simulink library "tqd"  (R2021b)
settings: Solver=VariableStepAuto  StartTime=0.0  StopTime=10.0  RelTol=1e-3
undefined symbols (not defined in the file): ATQD_AfterTqMinGain_X_Deg, ATQD_APSCreepBaseTqD_X_kph, ATQD_APSCreepBaseTqD_Y_Deg, ATQD_APSCreepBaseTqR_X_kph, ATQD_APSCreepBaseTqR_Y_Deg, ATQD_APSCreepIterm_X_kph, ATQD_APSCreepIterm_Y_kph, ATQD_APSCreepPterm_X_kph, ATQD_APSCreepPterm_Y_kph, ATQD_APSDecReq_X_kph, ATQD_APSDecReq_Y_mps2, ATQD_APSDecReqCMD_X_kph, ATQD_APSDecReqTs_X_pct, ATQD_APSDecTimeGain_X_Deg, ATQD_APSDecTimeGain_Y_s, ATQD_APSReqLowSpd_X_Deg, ATQD_AutoHoldReleaseBPS_X_Deg, ATQD_AWDLoadTrqnsGain_X_kg, ATQD_AWDLoadTrqnsGain_Y_pct, ATQD_BOSEnBPSPosn_X_kph, ATQD_BOSMap_X_rpm, ATQD_BOSMap_Y_pct, ATQD_CreepBaseTqD_X_kph, ATQD_CreepBaseTqD_Y_Deg, ATQD_CreepBaseTqR_X_kph, ATQD_CreepBaseTqR_Y_Deg, ATQD_CreepBPSDisPosn_X_Deg, ATQD_CreepBPSDisPosnR_X_Deg, ATQD_CreepBPSEnPosn_X_Deg, ATQD_CreepBPSEnPosnR_X_Deg, ATQD_CreepDeltaTq_X_kph, ATQD_CreepIterm_X_kph, ATQD_CreepIterm_Y_kph, ATQD_CreepItermMaxLimit_X_pct, ATQD_CreepPreloadTime_X_kph, ATQD_CreepPreloadTq_X_kph, ATQD_CreepPreloadTq_Y_s, ATQD_CreepProtTq_X_Deg, ATQD_CreepPterm_X_kph, ATQD_CreepPterm_Y_kph, ATQD_CreepRrTqSpRat_X_rpm, ATQD_CreepRrTqSpRat_Y_Nm, ATQD_CreepTargetSpdD_X_pct, ATQD_CreepTargetSpdR_X_pct, ATQD_ECOTqMapD_X_rpm, ATQD_ECOTqMapD_Y_pct, ATQD_EMTqMapD_X_rpm, ATQD_EMTqMapD_Y_pct, ATQD_EOPDTqMapDCon_X_rpm, ATQD_EOPDTqMapDCon_Y_Deg, ATQD_EscapeModePedTq_X_pct, ATQD_EscapeModePedTq_Y_rpm, ATQD_EscapeModePedTqFr_X_pct, ATQD_EscapeModePedTqFr_Y_rpm, ATQD_EstInitVehWeight_X_c, ATQD_FAfterTqCMDGain_X_rpm, ATQD_FAfterTqCMDGain_Y_pct, ATQD_FrLossMAPLowV_X_rpm, ATQD_FrLossMAPLowV_Y_Nm, ATQD_FrMotActReduce_X_rpm ... (+772)
libraries: simulink x211, hcu_lib x179, tqr x3
(part 20 of 28)

== system tqd/TQD/TorqueDemand/Signal_convert/SWC2_Subsystem/Big Mike Combo/Combo Key Detection/Engineering Mode ==
  note: Engineering Mode:
      | 5 = VINP_SWC2RScrollUpSta_flg
      | 5 = VINP_SWC2RScrollUpSta_flg
      | 6 = VINP_SWC2RScrollDownSta_flg
      | 6 = VINP_SWC2RScrollDownSta_flg
      | 5 = VINP_SWC2RScrollUpSta_flg
      | 6 = VINP_SWC2RScrollDownSta_flg
      | 5 = VINP_SWC2RScrollUpSta_flg
      | 6 = VINP_SWC2RScrollDownSta_flg
  TASK_TIME_10_MS : Inport
  VSCP_ComboKeyEn_flg : Inport  Port=2
  VSCP_ComboKeyReset_flg : Inport  Port=3
  VSCP_ComboKey_enum : Inport  Port=4
  VSCP_ComboKeyEnter_flg : Inport  Port=5
  VSCP_StreetFightModeOff_flg : Inport  Port=6
  AND : Logic  Inputs=9  AllPortsSameDT=off  OutDataTypeStr=boolean
  Constant : Constant  Value=ENUM_COMBOKEY_NONE
  Constant1 : Constant  Value=ENUM_COMBOKEY_NONE
  Constant2 : Constant  Value=FALSE
  Constant3 : Constant  Value=KTQD_ComboKeyDelay_s
  Delay : Delay  DelayLength=1
  DelayEnable : hcu_lib/Basic_Blocks/DelayEnable
  Equal : RelationalOperator  Operator=~=  OutDataTypeStr=boolean  RndMeth=Simplest
  Key1 : Subsystem
  Key2 : Subsystem
  Key3 : Subsystem
  Key4 : Subsystem
  Key5 : Subsystem
  Key6 : Subsystem
  Key7 : Subsystem
  Key8 : Subsystem
  Switch : Switch  Criteria=u2 > Threshold
  Switch1 : Switch  Criteria=u2 > Threshold
  Switch2 : Switch  Criteria=u2 > Threshold
  VSCP_EngineeringMode_flg : Outport
  wires:
  [VSCP_EngineeringMode_flg] -> VSCP_EngineeringMode_flg/1
  Switch/1 -> [VSCP_ComboKeyCMD_enum]  "VTQD_EngineeringCMD_enum"
  [TASK_TIME_10_MS] -> DelayEnable/3
  Constant/1 -> Switch/3
  DelayEnable/1 -> Switch/2
  [VSCP_ComboKeyEn_flg] -> DelayEnable/1
  Constant3/1 -> DelayEnable/2
  [VSCP_ComboKey_enum] -> Switch/1
  [VSCP_ComboKeyCMD_enum] -> Key1/1(VSCP_ComboKeyCMD_enum)
  [VSCP_ComboKeyEn_flg] -> Key1/2(VSCP_ComboKeyEn_flg)
  [VSCP_ComboKeyReset_flg] -> Key1/3(VSCP_ComboKeyReset_flg)
  [VSCP_ComboKeyCMD_enum] -> Key2/1(VSCP_ComboKeyCMD_enum)
  [VSCP_ComboKeyEn_flg] -> Key2/2(VSCP_ComboKeyEn_flg)
  [VSCP_ComboKeyReset_flg] -> Key2/3(VSCP_ComboKeyReset_flg)
  [VSCP_ComboKey1_enum] -> Key2/4(VSCP_ComboKey1_enum)
  Key1/1(VSCP_ComboKey1_enum) -> [VSCP_ComboKey1_enum]
  Key1/2(VSCP_Key1Pass_flg) -> [VSCP_Key1Pass_flg]
  [VSCP_ComboKeyCMD_enum] -> Key3/1(VSCP_ComboKeyCMD_enum)
  [VSCP_ComboKeyEn_flg] -> Key3/2(VSCP_ComboKeyEn_flg)
  [VSCP_ComboKeyReset_flg] -> Key3/3(VSCP_ComboKeyReset_flg)
  [VSCP_ComboKey2_enum] -> Key3/4(VSCP_ComboKey2_enum)
  [VSCP_ComboKeyCMD_enum] -> Key4/1(VSCP_ComboKeyCMD_enum)
  [VSCP_ComboKeyEn_flg] -> Key4/2(VSCP_ComboKeyEn_flg)
  [VSCP_ComboKeyReset_flg] -> Key4/3(VSCP_ComboKeyReset_flg)
  Key2/1(VSCP_ComboKey2_enum) -> [VSCP_ComboKey2_enum]
  Key2/2(VSCP_Key2Pass_flg) -> [VSCP_Key2Pass_flg]
  [VSCP_ComboKey3_enum] -> Key4/4(VSCP_ComboKey3_enum)
  Key3/1(VSCP_ComboKey3_enum) -> [VSCP_ComboKey3_enum]
  Key3/2(VSCP_Key3Pass_flg) -> [VSCP_Key3Pass_flg]
  Key4/1(VSCP_ComboKey4_enum) -> [VSCP_ComboKey4_enum]
  Key4/2(VSCP_Key4Pass_flg) -> [VSCP_Key4Pass_flg]
  [VSCP_ComboKeyReset_flg] -> Key5/3(VSCP_ComboKeyReset_flg)
  [VSCP_ComboKeyEn_flg] -> Key5/2(VSCP_ComboKeyEn_flg)
  [VSCP_ComboKeyCMD_enum] -> Key5/1(VSCP_ComboKeyCMD_enum)
  [VSCP_ComboKey4_enum] -> Key5/4(VSCP_ComboKey4_enum)
  Key5/2(VSCP_Key5Pass_flg) -> [VSCP_Key5Pass_flg]
  Key5/1(VSCP_ComboKey5_enum) -> [VSCP_ComboKey5_enum]
  Key7/2(VSCP_Key7Pass_flg) -> [VSCP_Key7Pass_flg]
  Key8/1(VSCP_ComboKey8_enum) -> [VSCP_ComboKey8_enum]
  Key8/2(VSCP_Key8Pass_flg) -> [VSCP_Key8Pass_flg]
  [VSCP_ComboKeyCMD_enum] -> Key6/1(VSCP_ComboKeyCMD_enum)
  [VSCP_ComboKeyEn_flg] -> Key6/2(VSCP_ComboKeyEn_flg)
  [VSCP_ComboKeyReset_flg] -> Key6/3(VSCP_ComboKeyReset_flg)
  [VSCP_ComboKey5_enum] -> Key6/4(VSCP_ComboKey5_enum)
  [VSCP_ComboKeyCMD_enum] -> Key7/1(VSCP_ComboKeyCMD_enum)
  [VSCP_ComboKeyEn_flg] -> Key7/2(VSCP_ComboKeyEn_flg)
  [VSCP_ComboKeyReset_flg] -> Key7/3(VSCP_ComboKeyReset_flg)
  [VSCP_ComboKey6_enum] -> Key7/4(VSCP_ComboKey6_enum)
  [VSCP_ComboKeyCMD_enum] -> Key8/1(VSCP_ComboKeyCMD_enum)
  [VSCP_ComboKeyEn_flg] -> Key8/2(VSCP_ComboKeyEn_flg)
  [VSCP_ComboKeyReset_flg] -> Key8/3(VSCP_ComboKeyReset_flg)
  [VSCP_ComboKey7_enum] -> Key8/4(VSCP_ComboKey7_enum)
  Constant1/1 -> Equal/2
  Equal/1 -> AND/1
  [VSCP_Key1Pass_flg] -> AND/2
  [VSCP_Key8Pass_flg] -> AND/9
  [VSCP_Key7Pass_flg] -> AND/8
  [VSCP_Key6Pass_flg] -> AND/7
  [VSCP_Key5Pass_flg] -> AND/6
  [VSCP_Key4Pass_flg] -> AND/5
  [VSCP_Key3Pass_flg] -> AND/4
  [VSCP_Key2Pass_flg] -> AND/3
  [VSCP_ComboKeyEnter_flg] -> Switch1/2
  AND/1 -> Switch1/1  "VTQD_EngineeringPass_flg"
  Switch1/1 -> Switch2/3
  [VSCP_StreetFightModeOff_flg] -> Switch2/2
  Constant2/1 -> Switch2/1
  Switch2/1 -> Delay/1, [VSCP_EngineeringMode_flg]  "VTQD_EngineeringMode_flg"
  Delay/1 -> Switch1/3
  TASK_TIME_10_MS/1 -> [TASK_TIME_10_MS]
  VSCP_ComboKeyEn_flg/1 -> [VSCP_ComboKeyEn_flg]
  VSCP_ComboKeyReset_flg/1 -> [VSCP_ComboKeyReset_flg]
  VSCP_ComboKey_enum/1 -> [VSCP_ComboKey_enum]
  VSCP_ComboKeyEnter_flg/1 -> [VSCP_ComboKeyEnter_flg]
  VSCP_StreetFightModeOff_flg/1 -> [VSCP_StreetFightModeOff_flg]
  Key6/1(VSCP_ComboKey6_enum) -> [VSCP_ComboKey6_enum]
  Key6/2(VSCP_Key6Pass_flg) -> [VSCP_Key6Pass_flg]
  Key7/1(VSCP_ComboKey7_enum) -> [VSCP_ComboKey7_enum]
  [VSCP_ComboKey8_enum] -> Equal/1

== system tqd/TQD/TorqueDemand/Signal_convert/SWC2_Subsystem/Big Mike Combo/Combo Key Detection/Exhibition Mode ==
  note: Exhibition Mode:
      | 7 = VINP_SWC2LScrollPressSta_flg
      | 7 = VINP_SWC2LScrollPressSta_flg
      | 8 = VINP_SWC2LADASSta_flg
      | 8 = VINP_SWC2LADASSta_flg
      | 8 = VINP_SWC2LADASSta_flg
      | 7 = VINP_SWC2LScrollPressSta_flg
      | 8 = VINP_SWC2LADASSta_flg
      | 7 = VINP_SWC2LScrollPressSta_flg
  TASK_TIME_10_MS : Inport
  VSCP_ComboKeyEn_flg : Inport  Port=2
  VSCP_ComboKeyReset_flg : Inport  Port=3
  VSCP_ComboKey_enum : Inport  Port=4
  VSCP_ComboKeyEnter_flg : Inport  Port=5
  VSCP_StreetFightModeOff_flg : Inport  Port=6
  AND : Logic  Inputs=9  AllPortsSameDT=off  OutDataTypeStr=boolean
  Constant : Constant  Value=ENUM_COMBOKEY_NONE
  Constant1 : Constant  Value=ENUM_COMBOKEY_NONE
  Constant2 : Constant  Value=FALSE
  Constant3 : Constant  Value=KTQD_ComboKeyDelay_s
  Delay : Delay  DelayLength=1
  DelayEnable : hcu_lib/Basic_Blocks/DelayEnable
  Equal : RelationalOperator  Operator=~=  OutDataTypeStr=boolean  RndMeth=Simplest
  Key1 : Subsystem
  Key2 : Subsystem
  Key3 : Subsystem
  Key4 : Subsystem
  Key5 : Subsystem
  Key6 : Subsystem
  Key7 : Subsystem
  Key8 : Subsystem
  Switch : Switch  Criteria=u2 > Threshold
  Switch1 : Switch  Criteria=u2 > Threshold
  Switch2 : Switch  Criteria=u2 > Threshold
  VSCP_ExhibitionMode_flg : Outport
  wires:
  [VSCP_ExhibitionMode_flg] -> VSCP_ExhibitionMode_flg/1
  Switch/1 -> [VSCP_ComboKeyCMD_enum]  "VTQD_ExhibitionCMD_enum"
  [TASK_TIME_10_MS] -> DelayEnable/3
  Constant/1 -> Switch/3
  DelayEnable/1 -> Switch/2
  [VSCP_ComboKeyEn_flg] -> DelayEnable/1
  Constant3/1 -> DelayEnable/2
  [VSCP_ComboKey_enum] -> Switch/1
  [VSCP_ComboKeyCMD_enum] -> Key1/1(VSCP_ComboKeyCMD_enum)
  [VSCP_ComboKeyEn_flg] -> Key1/2(VSCP_ComboKeyEn_flg)
  [VSCP_ComboKeyReset_flg] -> Key1/3(VSCP_ComboKeyReset_flg)
  [VSCP_ComboKeyCMD_enum] -> Key2/1(VSCP_ComboKeyCMD_enum)
  [VSCP_ComboKeyEn_flg] -> Key2/2(VSCP_ComboKeyEn_flg)
  [VSCP_ComboKeyReset_flg] -> Key2/3(VSCP_ComboKeyReset_flg)
  [VSCP_ComboKey1_enum] -> Key2/4(VSCP_ComboKey1_enum)
  Key1/1(VSCP_ComboKey1_enum) -> [VSCP_ComboKey1_enum]
  Key1/2(VSCP_Key1Pass_flg) -> [VSCP_Key1Pass_flg]
  [VSCP_ComboKeyCMD_enum] -> Key3/1(VSCP_ComboKeyCMD_enum)
  [VSCP_ComboKeyEn_flg] -> Key3/2(VSCP_ComboKeyEn_flg)
  [VSCP_ComboKeyReset_flg] -> Key3/3(VSCP_ComboKeyReset_flg)
  [VSCP_ComboKey2_enum] -> Key3/4(VSCP_ComboKey2_enum)
  [VSCP_ComboKeyCMD_enum] -> Key4/1(VSCP_ComboKeyCMD_enum)
  [VSCP_ComboKeyEn_flg] -> Key4/2(VSCP_ComboKeyEn_flg)
  [VSCP_ComboKeyReset_flg] -> Key4/3(VSCP_ComboKeyReset_flg)
  Key2/1(VSCP_ComboKey2_enum) -> [VSCP_ComboKey2_enum]
  Key2/2(VSCP_Key2Pass_flg) -> [VSCP_Key2Pass_flg]
  [VSCP_ComboKey3_enum] -> Key4/4(VSCP_ComboKey3_enum)
  Key3/1(VSCP_ComboKey3_enum) -> [VSCP_ComboKey3_enum]
  Key3/2(VSCP_Key3Pass_flg) -> [VSCP_Key3Pass_flg]
  Key4/1(VSCP_ComboKey4_enum) -> [VSCP_ComboKey4_enum]
  Key4/2(VSCP_Key4Pass_flg) -> [VSCP_Key4Pass_flg]
  [VSCP_ComboKeyReset_flg] -> Key5/3(VSCP_ComboKeyReset_flg)
  [VSCP_ComboKeyEn_flg] -> Key5/2(VSCP_ComboKeyEn_flg)
  [VSCP_ComboKeyCMD_enum] -> Key5/1(VSCP_ComboKeyCMD_enum)
  [VSCP_ComboKey4_enum] -> Key5/4(VSCP_ComboKey4_enum)
  Key5/2(VSCP_Key5Pass_flg) -> [VSCP_Key5Pass_flg]
  Key5/1(VSCP_ComboKey5_enum) -> [VSCP_ComboKey5_enum]
  Key7/2(VSCP_Key7Pass_flg) -> [VSCP_Key7Pass_flg]
  Key8/1(VSCP_ComboKey8_enum) -> [VSCP_ComboKey8_enum]
  Key8/2(VSCP_Key8Pass_flg) -> [VSCP_Key8Pass_flg]
  [VSCP_ComboKeyCMD_enum] -> Key6/1(VSCP_ComboKeyCMD_enum)
  [VSCP_ComboKeyEn_flg] -> Key6/2(VSCP_ComboKeyEn_flg)
  [VSCP_ComboKeyReset_flg] -> Key6/3(VSCP_ComboKeyReset_flg)
  [VSCP_ComboKey5_enum] -> Key6/4(VSCP_ComboKey5_enum)
  [VSCP_ComboKeyCMD_enum] -> Key7/1(VSCP_ComboKeyCMD_enum)
  [VSCP_ComboKeyEn_flg] -> Key7/2(VSCP_ComboKeyEn_flg)
  [VSCP_ComboKeyReset_flg] -> Key7/3(VSCP_ComboKeyReset_flg)
  [VSCP_ComboKey6_enum] -> Key7/4(VSCP_ComboKey6_enum)
  [VSCP_ComboKeyCMD_enum] -> Key8/1(VSCP_ComboKeyCMD_enum)
  [VSCP_ComboKeyEn_flg] -> Key8/2(VSCP_ComboKeyEn_flg)
  [VSCP_ComboKeyReset_flg] -> Key8/3(VSCP_ComboKeyReset_flg)
  [VSCP_ComboKey7_enum] -> Key8/4(VSCP_ComboKey7_enum)
  Constant1/1 -> Equal/2
  Equal/1 -> AND/1
  [VSCP_Key1Pass_flg] -> AND/2
  [VSCP_Key8Pass_flg] -> AND/9
  [VSCP_Key7Pass_flg] -> AND/8
  [VSCP_Key6Pass_flg] -> AND/7
  [VSCP_Key5Pass_flg] -> AND/6
  [VSCP_Key4Pass_flg] -> AND/5
  [VSCP_Key3Pass_flg] -> AND/4
  [VSCP_Key2Pass_flg] -> AND/3
  [VSCP_ComboKeyEnter_flg] -> Switch1/2
  AND/1 -> Switch1/1  "VTQD_ExhibitionPass_flg"
  Switch1/1 -> Switch2/3
  [VSCP_StreetFightModeOff_flg] -> Switch2/2
  Constant2/1 -> Switch2/1
  Switch2/1 -> Delay/1, [VSCP_ExhibitionMode_flg]  "VTQD_ExhibitionMode_flg"
  Delay/1 -> Switch1/3
  TASK_TIME_10_MS/1 -> [TASK_TIME_10_MS]
  VSCP_ComboKeyEn_flg/1 -> [VSCP_ComboKeyEn_flg]
  VSCP_ComboKeyReset_flg/1 -> [VSCP_ComboKeyReset_flg]
  VSCP_ComboKey_enum/1 -> [VSCP_ComboKey_enum]
  VSCP_ComboKeyEnter_flg/1 -> [VSCP_ComboKeyEnter_flg]
  VSCP_StreetFightModeOff_flg/1 -> [VSCP_StreetFightModeOff_flg]
  Key6/1(VSCP_ComboKey6_enum) -> [VSCP_ComboKey6_enum]
  Key6/2(VSCP_Key6Pass_flg) -> [VSCP_Key6Pass_flg]
  Key7/1(VSCP_ComboKey7_enum) -> [VSCP_ComboKey7_enum]
  [VSCP_ComboKey8_enum] -> Equal/1

== system tqd/TQD/TorqueDemand/Signal_convert/SWC2_Subsystem/Big Mike Combo/Combo Key Detection/Manufacture Mode ==
  note: Manufacture Mode:
      | 11 = VINP_SWC2RRightSta_flg
      | 12 = VINP_SWC2RLeftSta_flg
      | 11 = VINP_SWC2RRightSta_flg
      | 12 = VINP_SWC2RLeftSta_flg
      | 11 = VINP_SWC2RRightSta_flg
      | 12 = VINP_SWC2RLeftSta_flg
      | 7 = VINP_SWC2LScrollPressSta_flg
      | 8 = VINP_SWC2LADASSta_flg
  TASK_TIME_10_MS : Inport
  VSCP_ComboKeyEn_flg : Inport  Port=2
  VSCP_ComboKeyReset_flg : Inport  Port=3
  VSCP_ComboKey_enum : Inport  Port=4
  VSCP_ComboKeyEnter_flg : Inport  Port=5
  VSCP_StreetFightModeOff_flg : Inport  Port=6
  AND : Logic  Inputs=9  AllPortsSameDT=off  OutDataTypeStr=boolean
  Constant : Constant  Value=ENUM_COMBOKEY_NONE
  Constant1 : Constant  Value=ENUM_COMBOKEY_NONE
  Constant2 : Constant  Value=FALSE
  Constant3 : Constant  Value=KTQD_ComboKeyDelay_s
  Delay : Delay  DelayLength=1
  DelayEnable : hcu_lib/Basic_Blocks/DelayEnable
  Equal : RelationalOperator  Operator=~=  OutDataTypeStr=boolean  RndMeth=Simplest
  Key1 : Subsystem
  Key2 : Subsystem
  Key3 : Subsystem
  Key4 : Subsystem
  Key5 : Subsystem
  Key6 : Subsystem
  Key7 : Subsystem
  Key8 : Subsystem
  Switch : Switch  Criteria=u2 > Threshold
  Switch1 : Switch  Criteria=u2 > Threshold
  Switch2 : Switch  Criteria=u2 > Threshold
  VSCP_ManufactureMode_flg : Outport
  wires:
  [VSCP_ComboKey8_enum] -> Equal/1
  Key7/1(VSCP_ComboKey7_enum) -> [VSCP_ComboKey7_enum]
  Key6/2(VSCP_Key6Pass_flg) -> [VSCP_Key6Pass_flg]
  Key6/1(VSCP_ComboKey6_enum) -> [VSCP_ComboKey6_enum]
  VSCP_StreetFightModeOff_flg/1 -> [VSCP_StreetFightModeOff_flg]
  VSCP_ComboKeyEnter_flg/1 -> [VSCP_ComboKeyEnter_flg]
  VSCP_ComboKey_enum/1 -> [VSCP_ComboKey_enum]
  VSCP_ComboKeyReset_flg/1 -> [VSCP_ComboKeyReset_flg]
  VSCP_ComboKeyEn_flg/1 -> [VSCP_ComboKeyEn_flg]
  TASK_TIME_10_MS/1 -> [TASK_TIME_10_MS]
  Delay/1 -> Switch1/3
  Switch2/1 -> [VSCP_ManufactureMode_flg], Delay/1  "VTQD_ManufactureMode_flg"
  Constant2/1 -> Switch2/1
  [VSCP_StreetFightModeOff_flg] -> Switch2/2
  Switch1/1 -> Switch2/3
  AND/1 -> Switch1/1  "VTQD_ManufacturePass_flg"
  [VSCP_ComboKeyEnter_flg] -> Switch1/2
  [VSCP_Key2Pass_flg] -> AND/3
  [VSCP_Key3Pass_flg] -> AND/4
  [VSCP_Key4Pass_flg] -> AND/5
  [VSCP_Key5Pass_flg] -> AND/6
  [VSCP_Key6Pass_flg] -> AND/7
  [VSCP_Key7Pass_flg] -> AND/8
  [VSCP_Key8Pass_flg] -> AND/9
  [VSCP_Key1Pass_flg] -> AND/2
  Equal/1 -> AND/1
  Constant1/1 -> Equal/2
  [VSCP_ComboKey7_enum] -> Key8/4(VSCP_ComboKey7_enum)
  [VSCP_ComboKeyReset_flg] -> Key8/3(VSCP_ComboKeyReset_flg)
  [VSCP_ComboKeyEn_flg] -> Key8/2(VSCP_ComboKeyEn_flg)
  [VSCP_ComboKeyCMD_enum] -> Key8/1(VSCP_ComboKeyCMD_enum)
  [VSCP_ComboKey6_enum] -> Key7/4(VSCP_ComboKey6_enum)
  [VSCP_ComboKeyReset_flg] -> Key7/3(VSCP_ComboKeyReset_flg)
  [VSCP_ComboKeyEn_flg] -> Key7/2(VSCP_ComboKeyEn_flg)
  [VSCP_ComboKeyCMD_enum] -> Key7/1(VSCP_ComboKeyCMD_enum)
  [VSCP_ComboKey5_enum] -> Key6/4(VSCP_ComboKey5_enum)
  [VSCP_ComboKeyReset_flg] -> Key6/3(VSCP_ComboKeyReset_flg)
  [VSCP_ComboKeyEn_flg] -> Key6/2(VSCP_ComboKeyEn_flg)
  [VSCP_ComboKeyCMD_enum] -> Key6/1(VSCP_ComboKeyCMD_enum)
  Key8/2(VSCP_Key8Pass_flg) -> [VSCP_Key8Pass_flg]
  Key8/1(VSCP_ComboKey8_enum) -> [VSCP_ComboKey8_enum]
  Key7/2(VSCP_Key7Pass_flg) -> [VSCP_Key7Pass_flg]
  Key5/1(VSCP_ComboKey5_enum) -> [VSCP_ComboKey5_enum]
  Key5/2(VSCP_Key5Pass_flg) -> [VSCP_Key5Pass_flg]
  [VSCP_ComboKey4_enum] -> Key5/4(VSCP_ComboKey4_enum)
  [VSCP_ComboKeyCMD_enum] -> Key5/1(VSCP_ComboKeyCMD_enum)
  [VSCP_ComboKeyEn_flg] -> Key5/2(VSCP_ComboKeyEn_flg)
  [VSCP_ComboKeyReset_flg] -> Key5/3(VSCP_ComboKeyReset_flg)
  Key4/2(VSCP_Key4Pass_flg) -> [VSCP_Key4Pass_flg]
  Key4/1(VSCP_ComboKey4_enum) -> [VSCP_ComboKey4_enum]
  Key3/2(VSCP_Key3Pass_flg) -> [VSCP_Key3Pass_flg]
  Key3/1(VSCP_ComboKey3_enum) -> [VSCP_ComboKey3_enum]
  [VSCP_ComboKey3_enum] -> Key4/4(VSCP_ComboKey3_enum)
  Key2/2(VSCP_Key2Pass_flg) -> [VSCP_Key2Pass_flg]
  Key2/1(VSCP_ComboKey2_enum) -> [VSCP_ComboKey2_enum]
  [VSCP_ComboKeyReset_flg] -> Key4/3(VSCP_ComboKeyReset_flg)
  [VSCP_ComboKeyEn_flg] -> Key4/2(VSCP_ComboKeyEn_flg)
  [VSCP_ComboKeyCMD_enum] -> Key4/1(VSCP_ComboKeyCMD_enum)
  [VSCP_ComboKey2_enum] -> Key3/4(VSCP_ComboKey2_enum)
  [VSCP_ComboKeyReset_flg] -> Key3/3(VSCP_ComboKeyReset_flg)
  [VSCP_ComboKeyEn_flg] -> Key3/2(VSCP_ComboKeyEn_flg)
  [VSCP_ComboKeyCMD_enum] -> Key3/1(VSCP_ComboKeyCMD_enum)
  Key1/2(VSCP_Key1Pass_flg) -> [VSCP_Key1Pass_flg]
  Key1/1(VSCP_ComboKey1_enum) -> [VSCP_ComboKey1_enum]
  [VSCP_ComboKey1_enum] -> Key2/4(VSCP_ComboKey1_enum)
  [VSCP_ComboKeyReset_flg] -> Key2/3(VSCP_ComboKeyReset_flg)
  [VSCP_ComboKeyEn_flg] -> Key2/2(VSCP_ComboKeyEn_flg)
  [VSCP_ComboKeyCMD_enum] -> Key2/1(VSCP_ComboKeyCMD_enum)
  [VSCP_ComboKeyReset_flg] -> Key1/3(VSCP_ComboKeyReset_flg)
  [VSCP_ComboKeyEn_flg] -> Key1/2(VSCP_ComboKeyEn_flg)
  [VSCP_ComboKeyCMD_enum] -> Key1/1(VSCP_ComboKeyCMD_enum)
  [VSCP_ComboKey_enum] -> Switch/1
  Constant3/1 -> DelayEnable/2
  [VSCP_ComboKeyEn_flg] -> DelayEnable/1
  DelayEnable/1 -> Switch/2
  Constant/1 -> Switch/3
  [TASK_TIME_10_MS] -> DelayEnable/3
  Switch/1 -> [VSCP_ComboKeyCMD_enum]  "VTQD_ManufactureCMD_enum"
  [VSCP_ManufactureMode_flg] -> VSCP_ManufactureMode_flg/1

== system tqd/TQD/TorqueDemand/Signal_convert/SWC2_Subsystem/Big Mike Combo/Combo Key Detection/Street Fight Mode ==
  note: Street Fight Mode:
      | 3 = VINP_SWC2LScrollUpSta_flg
      | 3 = VINP_SWC2LScrollUpSta_flg
      | 4 = VINP_SWC2LScrollDownSta_flg
      | 4 = VINP_SWC2LScrollDownSta_flg
      | 1 = VINP_SWC2RegenDown_flg
      | 1 = VINP_SWC2RegenDown_flg
      | 2 = VINP_SWC2RegenUp_flg
      | 2 = VINP_SWC2RegenUp_flg
  TASK_TIME_10_MS : Inport
  VSCP_ComboKeyEn_flg : Inport  Port=2
  VSCP_ComboKeyReset_flg : Inport  Port=3
  VSCP_ComboKey_enum : Inport  Port=4
  VSCP_ComboKeyEnter_flg : Inport  Port=5
  VSCP_StreetFightModeOff_flg : Inport  Port=6
  AND : Logic  Inputs=9  AllPortsSameDT=off  OutDataTypeStr=boolean
  Constant : Constant  Value=ENUM_COMBOKEY_NONE
  Constant1 : Constant  Value=ENUM_COMBOKEY_NONE
  Constant2 : Constant  Value=FALSE
  Constant3 : Constant  Value=KTQD_ComboKeyDelay_s
  Delay : Delay  DelayLength=1
  DelayEnable : hcu_lib/Basic_Blocks/DelayEnable
  Equal : RelationalOperator  Operator=~=  OutDataTypeStr=boolean  RndMeth=Simplest
  Key1 : Subsystem
  Key2 : Subsystem
  Key3 : Subsystem
  Key4 : Subsystem
  Key5 : Subsystem
  Key6 : Subsystem
  Key7 : Subsystem
  Key8 : Subsystem
  Switch : Switch  Criteria=u2 > Threshold
  Switch1 : Switch  Criteria=u2 > Threshold
  Switch2 : Switch  Criteria=u2 > Threshold
  VSCP_StreetFightMode_flg : Outport
  wires:
  [VSCP_ComboKey8_enum] -> Equal/1
  Key7/1(VSCP_ComboKey7_enum) -> [VSCP_ComboKey7_enum]
  Key6/2(VSCP_Key6Pass_flg) -> [VSCP_Key6Pass_flg]
  Key6/1(VSCP_ComboKey6_enum) -> [VSCP_ComboKey6_enum]
  [VSCP_StreetFightMode_flg] -> VSCP_StreetFightMode_flg/1
  VSCP_StreetFightModeOff_flg/1 -> [VSCP_StreetFightModeOff_flg]
  VSCP_ComboKeyEnter_flg/1 -> [VSCP_ComboKeyEnter_flg]
  VSCP_ComboKey_enum/1 -> [VSCP_ComboKey_enum]
  VSCP_ComboKeyReset_flg/1 -> [VSCP_ComboKeyReset_flg]
  VSCP_ComboKeyEn_flg/1 -> [VSCP_ComboKeyEn_flg]
  TASK_TIME_10_MS/1 -> [TASK_TIME_10_MS]
  Delay/1 -> Switch1/3
  Switch2/1 -> [VSCP_StreetFightMode_flg], Delay/1  "VTQD_StreetFightMode_flg"
  Constant2/1 -> Switch2/1
  [VSCP_StreetFightModeOff_flg] -> Switch2/2
  Switch1/1 -> Switch2/3
  AND/1 -> Switch1/1  "VTQD_StreetFightPass_flg"
  [VSCP_ComboKeyEnter_flg] -> Switch1/2
  [VSCP_Key2Pass_flg] -> AND/3
  [VSCP_Key3Pass_flg] -> AND/4
  [VSCP_Key4Pass_flg] -> AND/5
  [VSCP_Key5Pass_flg] -> AND/6
  [VSCP_Key6Pass_flg] -> AND/7
  [VSCP_Key7Pass_flg] -> AND/8
  [VSCP_Key8Pass_flg] -> AND/9
  [VSCP_Key1Pass_flg] -> AND/2
  Equal/1 -> AND/1
  Constant1/1 -> Equal/2
  [VSCP_ComboKey7_enum] -> Key8/4(VSCP_ComboKey7_enum)
  [VSCP_ComboKeyReset_flg] -> Key8/3(VSCP_ComboKeyReset_flg)
  [VSCP_ComboKeyEn_flg] -> Key8/2(VSCP_ComboKeyEn_flg)
  [VSCP_ComboKeyCMD_enum] -> Key8/1(VSCP_ComboKeyCMD_enum)
  [VSCP_ComboKey6_enum] -> Key7/4(VSCP_ComboKey6_enum)
  [VSCP_ComboKeyReset_flg] -> Key7/3(VSCP_ComboKeyReset_flg)
  [VSCP_ComboKeyEn_flg] -> Key7/2(VSCP_ComboKeyEn_flg)
  [VSCP_ComboKeyCMD_enum] -> Key7/1(VSCP_ComboKeyCMD_enum)
  [VSCP_ComboKey5_enum] -> Key6/4(VSCP_ComboKey5_enum)
  [VSCP_ComboKeyReset_flg] -> Key6/3(VSCP_ComboKeyReset_flg)
  [VSCP_ComboKeyEn_flg] -> Key6/2(VSCP_ComboKeyEn_flg)
  [VSCP_ComboKeyCMD_enum] -> Key6/1(VSCP_ComboKeyCMD_enum)
  Key8/2(VSCP_Key8Pass_flg) -> [VSCP_Key8Pass_flg]
  Key8/1(VSCP_ComboKey8_enum) -> [VSCP_ComboKey8_enum]
  Key7/2(VSCP_Key7Pass_flg) -> [VSCP_Key7Pass_flg]
  Key5/1(VSCP_ComboKey5_enum) -> [VSCP_ComboKey5_enum]
  Key5/2(VSCP_Key5Pass_flg) -> [VSCP_Key5Pass_flg]
  [VSCP_ComboKey4_enum] -> Key5/4(VSCP_ComboKey4_enum)
  [VSCP_ComboKeyCMD_enum] -> Key5/1(VSCP_ComboKeyCMD_enum)
  [VSCP_ComboKeyEn_flg] -> Key5/2(VSCP_ComboKeyEn_flg)
  [VSCP_ComboKeyReset_flg] -> Key5/3(VSCP_ComboKeyReset_flg)
  Key4/2(VSCP_Key4Pass_flg) -> [VSCP_Key4Pass_flg]
  Key4/1(VSCP_ComboKey4_enum) -> [VSCP_ComboKey4_enum]
  Key3/2(VSCP_Key3Pass_flg) -> [VSCP_Key3Pass_flg]
  Key3/1(VSCP_ComboKey3_enum) -> [VSCP_ComboKey3_enum]
  [VSCP_ComboKey3_enum] -> Key4/4(VSCP_ComboKey3_enum)
  Key2/2(VSCP_Key2Pass_flg) -> [VSCP_Key2Pass_flg]
  Key2/1(VSCP_ComboKey2_enum) -> [VSCP_ComboKey2_enum]
  [VSCP_ComboKeyReset_flg] -> Key4/3(VSCP_ComboKeyReset_flg)
  [VSCP_ComboKeyEn_flg] -> Key4/2(VSCP_ComboKeyEn_flg)
  [VSCP_ComboKeyCMD_enum] -> Key4/1(VSCP_ComboKeyCMD_enum)
  [VSCP_ComboKey2_enum] -> Key3/4(VSCP_ComboKey2_enum)
  [VSCP_ComboKeyReset_flg] -> Key3/3(VSCP_ComboKeyReset_flg)
  [VSCP_ComboKeyEn_flg] -> Key3/2(VSCP_ComboKeyEn_flg)
  [VSCP_ComboKeyCMD_enum] -> Key3/1(VSCP_ComboKeyCMD_enum)
  Key1/2(VSCP_Key1Pass_flg) -> [VSCP_Key1Pass_flg]
  Key1/1(VSCP_ComboKey1_enum) -> [VSCP_ComboKey1_enum]
  [VSCP_ComboKey1_enum] -> Key2/4(VSCP_ComboKey1_enum)
  [VSCP_ComboKeyReset_flg] -> Key2/3(VSCP_ComboKeyReset_flg)
  [VSCP_ComboKeyEn_flg] -> Key2/2(VSCP_ComboKeyEn_flg)
  [VSCP_ComboKeyCMD_enum] -> Key2/1(VSCP_ComboKeyCMD_enum)
  [VSCP_ComboKeyReset_flg] -> Key1/3(VSCP_ComboKeyReset_flg)
  [VSCP_ComboKeyEn_flg] -> Key1/2(VSCP_ComboKeyEn_flg)
  [VSCP_ComboKeyCMD_enum] -> Key1/1(VSCP_ComboKeyCMD_enum)
  [VSCP_ComboKey_enum] -> Switch/1
  Constant3/1 -> DelayEnable/2
  [VSCP_ComboKeyEn_flg] -> DelayEnable/1
  DelayEnable/1 -> Switch/2
  Constant/1 -> Switch/3
  [TASK_TIME_10_MS] -> DelayEnable/3
  Switch/1 -> [VSCP_ComboKeyCMD_enum]  "VTQD_StreetFightCMD_enum"

== system tqd/TQD/TorqueDemand/Signal_convert/SWC2_Subsystem/Big Mike Combo/Mode Coordination/DiagnosisOff ==
  Action Port : ActionPort
  Constant : Constant  Value=ENUM_SYSMODE_DIAGNOSISOFF
  DiagnosisOff : Outport
  wires:
  Constant/1 -> DiagnosisOff/1

== system tqd/TQD/TorqueDemand/Signal_convert/SWC2_Subsystem/Big Mike Combo/Mode Coordination/Engineering ==
  Action Port : ActionPort
  Constant : Constant  Value=ENUM_SYSMODE_ENGINEERING
  Engineering : Outport
  wires:
  Constant/1 -> Engineering/1

== system tqd/TQD/TorqueDemand/Signal_convert/SWC2_Subsystem/Big Mike Combo/Mode Coordination/Exhibition ==
  Action Port : ActionPort
  Constant : Constant  Value=ENUM_SYSMODE_EXHIBITION
  Exhibition : Outport
  wires:
  Constant/1 -> Exhibition/1

== system tqd/TQD/TorqueDemand/Signal_convert/SWC2_Subsystem/Big Mike Combo/Mode Coordination/Manufacture ==
  Action Port : ActionPort
  Constant : Constant  Value=ENUM_SYSMODE_MANUFACTURE
  Manufacture : Outport
  wires:
  Constant/1 -> Manufacture/1

== system tqd/TQD/TorqueDemand/Signal_convert/SWC2_Subsystem/Big Mike Combo/Mode Coordination/Product ==
  Action Port : ActionPort
  Constant : Constant  Value=ENUM_SYSMODE_PRODUCT
  Product : Outport
  wires:
  Constant/1 -> Product/1

== system tqd/TQD/TorqueDemand/Signal_convert/SWC2_Subsystem/Big Mike Combo/Mode Coordination/StreetFight ==
  Action Port : ActionPort
  Constant : Constant  Value=ENUM_SYSMODE_DEVELOPING
  StreetFight : Outport
  wires:
  Constant/1 -> StreetFight/1

== system tqd/TQD/TorqueDemand/Signal_convert/SWC2_Subsystem/Big Mike Combo/Signal Status Detection/None ==
  Action Port : ActionPort
  Constant : Constant  Value=ENUM_COMBOKEY_NONE  OutDataTypeStr=uint8
  None_enum : Outport
  wires:
  Constant/1 -> None_enum/1

== system tqd/TQD/TorqueDemand/Signal_convert/SWC2_Subsystem/Big Mike Combo/Signal Status Detection/SWCACCSta ==
  Action Port : ActionPort
  Constant : Constant  Value=ENUM_COMBOKEY_SWCACC  OutDataTypeStr=uint8
  SWCACCSta_enum : Outport
  wires:
  Constant/1 -> SWCACCSta_enum/1

== system tqd/TQD/TorqueDemand/Signal_convert/SWC2_Subsystem/Big Mike Combo/Signal Status Detection/SWCCANCELStaShort ==
  Action Port : ActionPort
  Constant : Constant  Value=ENUM_COMBOKEY_CANCEL  OutDataTypeStr=uint8
  SWCCANCELStaShort_enum : Outport
  wires:
  Constant/1 -> SWCCANCELStaShort_enum/1

== system tqd/TQD/TorqueDemand/Signal_convert/SWC2_Subsystem/Big Mike Combo/Signal Status Detection/SWCDistanceSta ==
  Action Port : ActionPort
  Constant : Constant  Value=ENUM_COMBOKEY_DISTANCE  OutDataTypeStr=uint8
  SWCDownStaShort_enum : Outport
  wires:
  Constant/1 -> SWCDownStaShort_enum/1

== system tqd/TQD/TorqueDemand/Signal_convert/SWC2_Subsystem/Big Mike Combo/Signal Status Detection/SWCDownStaShort ==
  Action Port : ActionPort
  Constant : Constant  Value=ENUM_COMBOKEY_SWCDOWN  OutDataTypeStr=uint8
  SWCDownStaShort_enum : Outport
  wires:
  Constant/1 -> SWCDownStaShort_enum/1

== system tqd/TQD/TorqueDemand/Signal_convert/SWC2_Subsystem/Big Mike Combo/Signal Status Detection/SWCLeftSta ==
  Action Port : ActionPort
  Constant : Constant  Value=ENUM_COMBOKEY_SWCLEFT  OutDataTypeStr=uint8
  SWCLeftSta_enum : Outport
  wires:
  Constant/1 -> SWCLeftSta_enum/1

== system tqd/TQD/TorqueDemand/Signal_convert/SWC2_Subsystem/Big Mike Combo/Signal Status Detection/SWCRegenDownShort ==
  Action Port : ActionPort
  Constant : Constant  Value=ENUM_COMBOKEY_REGENDOWN  OutDataTypeStr=uint8
  SWCRegenDownShort_enum : Outport
  wires:
  Constant/1 -> SWCRegenDownShort_enum/1

== system tqd/TQD/TorqueDemand/Signal_convert/SWC2_Subsystem/Big Mike Combo/Signal Status Detection/SWCRegenUpShort ==
  Action Port : ActionPort
  Constant : Constant  Value=ENUM_COMBOKEY_REGENUP  OutDataTypeStr=uint8
  SWCRegenUpShort_enum : Outport
  wires:
  Constant/1 -> SWCRegenUpShort_enum/1

== system tqd/TQD/TorqueDemand/Signal_convert/SWC2_Subsystem/Big Mike Combo/Signal Status Detection/SWCResUpStaShort ==
  Action Port : ActionPort
  Constant : Constant  Value=ENUM_COMBOKEY_RESUP  OutDataTypeStr=uint8
  SWCResUpStaShort_enum : Outport
  wires:
  Constant/1 -> SWCResUpStaShort_enum/1

== system tqd/TQD/TorqueDemand/Signal_convert/SWC2_Subsystem/Big Mike Combo/Signal Status Detection/SWCRightSta ==
  Action Port : ActionPort
  Constant : Constant  Value=ENUM_COMBOKEY_SWCRIGHT  OutDataTypeStr=uint8
  SWCRightSta_enum : Outport
  wires:
  Constant/1 -> SWCRightSta_enum/1

== system tqd/TQD/TorqueDemand/Signal_convert/SWC2_Subsystem/Big Mike Combo/Signal Status Detection/SWCSetdownStaShort ==
  Action Port : ActionPort
  Constant : Constant  Value=ENUM_COMBOKEY_SETDOWN  OutDataTypeStr=uint8
  SWCSetdownStaShort_enum : Outport
  wires:
  Constant/1 -> SWCSetdownStaShort_enum/1

== system tqd/TQD/TorqueDemand/Signal_convert/SWC2_Subsystem/Big Mike Combo/Signal Status Detection/SWCUpStaShort ==
  Action Port : ActionPort
  Constant : Constant  Value=ENUM_COMBOKEY_SWCUP  OutDataTypeStr=uint8
  SWCUpStaShort_enum : Outport
  wires:
  Constant/1 -> SWCUpStaShort_enum/1

== system tqd/TQD/TorqueDemand/Signal_convert/SWC2_Subsystem/Big Mike Combo/Signal Status Detection/SWCmodeSta ==
  Action Port : ActionPort
  Constant : Constant  Value=ENUM_COMBOKEY_SWCMODE  OutDataTypeStr=uint8
  SWCmodeSta_enum : Outport
  wires:
  Constant/1 -> SWCmodeSta_enum/1

== system tqd/TQD/TorqueDemand/Signal_convert/SWC2_Subsystem/Big Mike Combo/Signal Status Detection/Street Fight Switch Off ==
  TASK_TIME_10_MS : Inport
  VSCP_SWCCANCELStaShort_flg : Inport  Port=2
  VSCP_ComboKeyPreEn_flg : Inport  Port=3
  SWCCANCELStaLong_flg : Inport  Port=4
  VSCP_SysMode_enum : Inport  Port=5
  AND : Logic  AllPortsSameDT=off  OutDataTypeStr=boolean
  AND2 : Logic  AllPortsSameDT=off  OutDataTypeStr=boolean
  Add : Sum
  Constant1 : Constant  Value=ZERO_INT
  Constant11 : Constant  Value=ONE_INT
  Constant2 : Constant  Value=ONE_INT
  Constant3 : Constant  Value=KTQD_CANCELUpCount_cnt
  Constant4 : Constant  Value=ZERO_INT
  Constant5 : Constant  Value=ENUM_SYSMODE_PRODUCT
  Constant7 : Constant  Value=KTQD_CANCELCountDetTime_s
  Delay{,1..3} (4 alike) : Delay  DelayLength=1
  Equal : RelationalOperator  Operator===  OutDataTypeStr=boolean  RndMeth=Simplest
  Equal1 : RelationalOperator  Operator===  OutDataTypeStr=boolean  RndMeth=Simplest
  Equal2 : RelationalOperator  Operator===  OutDataTypeStr=boolean  RndMeth=Simplest
  NOT : Logic  Operator=NOT  AllPortsSameDT=off  OutDataTypeStr=boolean
  NOT1 : Logic  Operator=NOT  AllPortsSameDT=off  OutDataTypeStr=boolean
  OR : Logic  Operator=OR  Inputs=3  AllPortsSameDT=off  OutDataTypeStr=boolean
  Relational Operator : RelationalOperator  OutDataTypeStr=boolean  RndMeth=Simplest
  SR_Latch : hcu_lib/Basic_Blocks/SR_Latch
  Switch : Switch  Criteria=u2 > Threshold
  Switch1 : Switch  Criteria=u2 > Threshold
  Timer : hcu_lib/Basic_Blocks/Timer
  VSCP_StreetFightModeOff_flg : Outport
  wires:
  Constant5/1 -> Equal2/1
  Delay3/1 -> Equal2/2
  [VSCP_SysMode_enum] -> Delay3/1
  [VSCP_CANCELCountReset_flg] -> Switch1/2
  OR/1 -> [VSCP_CANCELCountReset_flg]  "VTQD_CANCELCountReset_flg"
  Delay2/1 -> OR/3
  NOT1/1 -> OR/2
  Equal2/1 -> OR/1
  VSCP_SysMode_enum/1 -> [VSCP_SysMode_enum]
  [VSCP_ComboKeyPreEn_flg] -> NOT1/1
  [VSCP_StreetFightModeOff_flg] -> VSCP_StreetFightModeOff_flg/1
  SWCCANCELStaLong_flg/1 -> [SWCCANCELStaLong_flg]
  VSCP_ComboKeyPreEn_flg/1 -> [VSCP_ComboKeyPreEn_flg]
  VSCP_SWCCANCELStaShort_flg/1 -> [VSCP_SWCCANCELStaShort_flg]
  TASK_TIME_10_MS/1 -> [TASK_TIME_10_MS]
  AND2/1 -> [VSCP_StreetFightModeOff_flg]  "VTQD_StreetFightModeOff_flg"
  Equal1/1 -> AND2/1
  Constant4/1 -> Switch1/1
  [VSCP_CANCELCountDetFinish_flg] -> Delay2/1
  Delay1/1 -> SR_Latch/2
  [VSCP_CANCELCountDetFinish_flg] -> Delay1/1
  [SWCCANCELStaLong_flg] -> AND2/2
  Constant3/1 -> Equal1/2
  [VSCP_CANCELCount_cnt] -> Equal1/1
  Relational Operator/1 -> [VSCP_CANCELCountDetFinish_flg]  "VTQD_CANCELCountDetFinish_flg"
  Timer/1 -> Relational Operator/1  "VTQD_CANCELCountDetTime_s"
  Constant7/1 -> Timer/4, Relational Operator/2
  [TASK_TIME_10_MS] -> Timer/3
  NOT/1 -> Timer/2
  SR_Latch/1 -> Timer/1, NOT/1
  AND/1 -> SR_Latch/1
  [VSCP_ComboKeyPreEn_flg] -> AND/2
  Equal/1 -> AND/1
  Constant2/1 -> Equal/2
  [VSCP_CANCELCount_cnt] -> Equal/1
  Delay/1 -> Add/2
  Switch1/1 -> Delay/1, [VSCP_CANCELCount_cnt]  "VTQD_CANCELCount_cnt"
  Add/1 -> Switch1/3
  Switch/1 -> Add/1
  Constant11/1 -> Switch/1
  [VSCP_SWCCANCELStaShort_flg] -> Switch/2
  Constant1/1 -> Switch/3

== system tqd/TQD/TorqueDemand/TorqueModule/DriverWhlTqDem/PedalMapWhlTq/NoLHM/ShiftD ==
  VTQD_EVDriveMode_enum : Inport
  VTQD_ActAPSPosn_pct : Inport  Port=2
  VTQD_TqTargetShaftSpd_rpm : Inport  Port=3
  VTQD_RegenMode_enum : Inport  Port=4
  VTQD_RollRegenEnable_flg : Inport  Port=5
  VTQD_RollingShaftSpd_rpm : Inport  Port=6
  VVMC_EstSlope_Deg : Inport  Port=7
  VTQD_APSReqTimer_s : Inport  Port=8
  VTQD_LowIdleAccPedal_flg : Inport  Port=9
  VTQD_OPDHoldEnRel_flg : Inport  Port=10
  VTQD_OPDHoldActRelTq_Nm : Inport  Port=11
  VTQD_VehActSpd_kph : Inport  Port=12
  VTQD_SlopeUp_flg : Inport  Port=13
  VINP_IVISnowModeCmd_flg : Inport  Port=14
  VTQD_IVIRockModeEn_flg : Inport  Port=15
  VTQD_PreDecTqLowLim_Nm : Inport  Port=16
  VTQD_BrkSwSta_flg : Inport  Port=17
  VTQD_CreepEnable_flg : Inport  Port=18
  Action Port : ActionPort
  AND{,1..4} (5 alike) : Logic  AllPortsSameDT=off  OutDataTypeStr=boolean
  Bus Creator : BusCreator  Inputs=5
  Constant{,1..4} (5 alike) : Constant  Value=ZERO_FLOAT
  Constant5 : Constant  Value=ENUM_DRIVEMODE_NRM
  Constant6 : Constant  Value=ENUM_DRIVEMODE_ECO
  Constant7 : Constant  Value=ENUM_DRIVEMODE_SPORT
  Delay{,1..4} (5 alike) : Delay  DelayLength=1
  Equal1 : RelationalOperator  Operator===  OutDataTypeStr=boolean  RndMeth=Simplest
  Equal2 : RelationalOperator  Operator===  OutDataTypeStr=boolean  RndMeth=Simplest
  Equal3 : RelationalOperator  Operator===  OutDataTypeStr=boolean  RndMeth=Simplest
  If : If  NumInputs=5  IfExpression=u1 ~= 0  ElseIfExpressions=u2 ~= 0, u3 ~= 0, u4 ~= 0
  LUT_D_ECO : Subsystem  TreatAsAtomicUnit=on
  LUT_D_EscapeMode : Subsystem  TreatAsAtomicUnit=on
  LUT_D_Normal : Subsystem  TreatAsAtomicUnit=on
  LUT_D_SnowMode : Subsystem  TreatAsAtomicUnit=on
  LUT_D_Sport : Subsystem  TreatAsAtomicUnit=on
  MTQD_RL1TqMapDComp_Z_Nm : Lookup_n-D  BreakpointsForDimension1=ATQD_RL1TqMapDComp_Y_Deg  BreakpointsForDimension2=ATQD_RL1TqMapDComp_X_rpm  Table=MTQD_RL1TqMapDComp_Z_Nm  ExtrapMethod=Clip  InternalRulePriority=Speed  RndMeth=Simplest  InputSameDT=on
      settings: InputPortMap=u0,u1
  MTQD_RL2TqMapDComp_Z_Nm : Lookup_n-D  BreakpointsForDimension1=ATQD_RL1TqMapDComp_Y_Deg  BreakpointsForDimension2=ATQD_RL1TqMapDComp_X_rpm  Table=MTQD_RL2TqMapDComp_Z_Nm  ExtrapMethod=Clip  InternalRulePriority=Speed  RndMeth=Simplest  InputSameDT=on
      settings: InputPortMap=u0,u1
  MTQD_RL3TqMapDComp_Z_Nm : Lookup_n-D  BreakpointsForDimension1=ATQD_RL1TqMapDComp_Y_Deg  BreakpointsForDimension2=ATQD_RL1TqMapDComp_X_rpm  Table=MTQD_RL3TqMapDComp_Z_Nm  ExtrapMethod=Clip  InternalRulePriority=Speed  RndMeth=Simplest  InputSameDT=on
      settings: InputPortMap=u0,u1
  MTQD_RL4TqMapDComp_Z_Nm : Lookup_n-D  BreakpointsForDimension1=ATQD_RL1TqMapDComp_Y_Deg  BreakpointsForDimension2=ATQD_RL1TqMapDComp_X_rpm  Table=MTQD_RL4TqMapDComp_Z_Nm  ExtrapMethod=Clip  InternalRulePriority=Speed  RndMeth=Simplest  InputSameDT=on
      settings: InputPortMap=u0,u1
  MTQD_RL5TqMapDComp_Z_Nm : Lookup_n-D  BreakpointsForDimension1=ATQD_RL1TqMapDComp_Y_Deg  BreakpointsForDimension2=ATQD_RL1TqMapDComp_X_rpm  Table=MTQD_RL5TqMapDComp_Z_Nm  ExtrapMethod=Clip  InternalRulePriority=Speed  RndMeth=Simplest  InputSameDT=on
      settings: InputPortMap=u0,u1
  Merge : Merge  Inputs=5
  NOT{,1..4} (5 alike) : Logic  Operator=NOT  AllPortsSameDT=off  OutDataTypeStr=boolean
  Switch{,1..4} (5 alike) : Switch  Criteria=u2 > Threshold
  VTQD_PedalMapWhlTqD_Nm : Outport
  wires:
  [VTQD_RollingShaftSpd_rpm] -> LUT_D_ECO/5(VTQD_RollingShaftSpd_rpm)
  [VTQD_RollRegenEnable_flg] -> LUT_D_ECO/4(VTQD_RollRegenEnable_flg)
  VTQD_RollingShaftSpd_rpm/1 -> [VTQD_RollingShaftSpd_rpm]
  VTQD_RollRegenEnable_flg/1 -> [VTQD_RollRegenEnable_flg]
  [VTQD_TqTargetShaftSpd_rpm] -> LUT_D_Sport/1(VTQD_TqTargetShaftSpd_rpm)
  [VTQD_ActAPSPosn_pct] -> LUT_D_Sport/2(VTQD_ActAPSPosn_pct)
  [VTQD_RegenMode_enum] -> LUT_D_Sport/3(VTQD_RegenMode_enum)
  [VTQD_RegenMode_enum] -> LUT_D_ECO/3(VTQD_RegenMode_enum)
  [VTQD_ActAPSPosn_pct] -> LUT_D_ECO/2(VTQD_ActAPSPosn_pct)
  [VTQD_TqTargetShaftSpd_rpm] -> LUT_D_ECO/1(VTQD_TqTargetShaftSpd_rpm)
  [VTQD_ActAPSPosn_pct] -> LUT_D_Normal/2(VTQD_ActAPSPosn_pct)
  [VTQD_TqTargetShaftSpd_rpm] -> LUT_D_Normal/1(VTQD_TqTargetShaftSpd_rpm)
  [VTQD_RegenMode_enum] -> LUT_D_Normal/3(VTQD_RegenMode_enum)
  VTQD_RegenMode_enum/1 -> [VTQD_RegenMode_enum]
  VTQD_TqTargetShaftSpd_rpm/1 -> [VTQD_TqTargetShaftSpd_rpm]
  VTQD_ActAPSPosn_pct/1 -> [VTQD_ActAPSPosn_pct]
  VTQD_EVDriveMode_enum/1 -> [VTQD_EVDriveMode_enum]
  Merge/1 -> VTQD_PedalMapWhlTqD_Nm/1
  Constant7/1 -> Equal3/2
  Constant5/1 -> Equal1/2
  [VTQD_EVDriveMode_enum] -> Equal3/1
  Constant6/1 -> Equal2/2
  [VTQD_EVDriveMode_enum] -> Equal2/1
  [VTQD_EVDriveMode_enum] -> Equal1/1
  [VVMC_EstSlope_Deg] -> LUT_D_Normal/4(VVMC_EstSlope_Deg)
  [VTQD_APSReqTimer_s] -> LUT_D_Normal/5(VTQD_APSReqTimer_s)
  VVMC_EstSlope_Deg/1 -> [VVMC_EstSlope_Deg]
  VTQD_APSReqTimer_s/1 -> [VTQD_APSReqTimer_s]
  [VVMC_EstSlope_Deg] -> LUT_D_ECO/6(VVMC_EstSlope_Deg)
  [VTQD_APSReqTimer_s] -> LUT_D_ECO/7(VTQD_APSReqTimer_s)
  [VVMC_EstSlope_Deg] -> LUT_D_Sport/4(VVMC_EstSlope_Deg)
  [VTQD_APSReqTimer_s] -> LUT_D_Sport/5(VTQD_APSReqTimer_s)
  [VTQD_LowIdleAccPedal_flg] -> LUT_D_Normal/6(VTQD_LowIdleAccPedal_flg)
  VTQD_LowIdleAccPedal_flg/1 -> [VTQD_LowIdleAccPedal_flg]
  [VTQD_LowIdleAccPedal_flg] -> LUT_D_ECO/8(VTQD_LowIdleAccPedal_flg)
  [VTQD_LowIdleAccPedal_flg] -> LUT_D_Sport/6(VTQD_LowIdleAccPedal_flg)
  VTQD_OPDHoldEnRel_flg/1 -> [VTQD_OPDHoldEnRel_flg]
  [VTQD_OPDHoldEnRel_flg] -> LUT_D_Normal/7(VTQD_OPDHoldEnRel_flg)
  VTQD_OPDHoldActRelTq_Nm/1 -> [VTQD_OPDHoldActRelTq_Nm]
  VTQD_VehActSpd_kph/1 -> [VTQD_VehActSpd_kph]
  [VTQD_VehActSpd_kph] -> LUT_D_Normal/9(VTQD_VehActSpd_kph)
  [VTQD_OPDHoldActRelTq_Nm] -> LUT_D_Normal/8(VTQD_OPDHoldActRelTq_Nm)
  [VTQD_OPDHoldEnRel_flg] -> LUT_D_ECO/9(VTQD_OPDHoldEnRel_flg)
  [VTQD_OPDHoldActRelTq_Nm] -> LUT_D_ECO/10(VTQD_OPDHoldActRelTq_Nm)
  [VTQD_VehActSpd_kph] -> LUT_D_ECO/11(VTQD_VehActSpd_kph)
  [VTQD_VehActSpd_kph] -> LUT_D_Sport/9(VTQD_VehActSpd_kph)
  [VTQD_OPDHoldActRelTq_Nm] -> LUT_D_Sport/8(VTQD_OPDHoldActRelTq_Nm)
  [VTQD_OPDHoldEnRel_flg] -> LUT_D_Sport/7(VTQD_OPDHoldEnRel_flg)
  VTQD_SlopeUp_flg/1 -> [VTQD_SlopeUp_flg]
  [VTQD_SlopeUp_flg] -> LUT_D_Normal/10(VTQD_SlopeUp_flg)
  [VTQD_SlopeUp_flg] -> LUT_D_Sport/10(VTQD_SlopeUp_flg)
  [VTQD_SlopeUp_flg] -> LUT_D_ECO/12(VTQD_SlopeUp_flg)
  VTQD_IVIRockModeEn_flg/1 -> [VTQD_IVIRockModeEn_flg]
  VINP_IVISnowModeCmd_flg/1 -> [VINP_IVISnowModeCmd_flg]
  Equal3/1 -> If/5
  Equal2/1 -> If/4
  Equal1/1 -> If/3
  If/4 -> LUT_D_ECO/Action
  If/5 -> LUT_D_Sport/Action
  If/3 -> LUT_D_Normal/Action
  [VTQD_IVIRockModeEn_flg] -> If/1
  [VINP_IVISnowModeCmd_flg] -> If/2
  [VTQD_RegenMode_enum] -> LUT_D_SnowMode/3(VTQD_RegenMode_enum)
  [VTQD_ActAPSPosn_pct] -> LUT_D_SnowMode/2(VTQD_ActAPSPosn_pct)
  [VTQD_TqTargetShaftSpd_rpm] -> LUT_D_SnowMode/1(VTQD_TqTargetShaftSpd_rpm)
  If/2 -> LUT_D_SnowMode/Action
  If/1 -> LUT_D_EscapeMode/Action
  [VTQD_TqTargetShaftSpd_rpm] -> LUT_D_EscapeMode/1(VTQD_TqTargetShaftSpd_rpm)
  [VTQD_ActAPSPosn_pct] -> LUT_D_EscapeMode/2(VTQD_ActAPSPosn_pct)
  LUT_D_EscapeMode/1(VTQD_WhlTqEscapeMode_Nm) -> [VTQD_WhlTqEscapeMode_Nm]  "VTQD_WhlTqEscapeMode_Nm"
  LUT_D_SnowMode/1(VTQD_WhlTqSnowMode_Nm) -> [VTQD_WhlTqSnowMode_Nm]  "VTQD_WhlTqSnowMode_Nm"
  LUT_D_Normal/1(VTQD_WhlTqNRMD_Nm) -> [VTQD_WhlTqNRMD_Nm]  "VTQD_WhlTqNRMD_Nm"
  LUT_D_ECO/1(VTQD_WhlTqECOD_Nm) -> [VTQD_WhlTqECOD_Nm]  "VTQD_WhlTqECOD_Nm"
  LUT_D_Sport/1(VTQD_WhlTqSPORTD_Nm) -> [VTQD_WhlTqSPORTD_Nm]  "VTQD_WhlTqSPORTD_Nm"
  [VTQD_WhlTqEscapeMode_Nm] -> Merge/1
  [VTQD_WhlTqSnowMode_Nm] -> Merge/2
  [VTQD_WhlTqNRMD_Nm] -> Merge/3
  [VTQD_WhlTqECOD_Nm] -> Merge/4
  [VTQD_WhlTqSPORTD_Nm] -> Merge/5
  [VTQD_PreDecTqLowLim_Nm] -> LUT_D_SnowMode/4(VTQD_PreDecTqLowLim_Nm)
  VTQD_PreDecTqLowLim_Nm/1 -> [VTQD_PreDecTqLowLim_Nm]
  [VTQD_TqTargetShaftSpd_rpm] -> MTQD_RL1TqMapDComp_Z_Nm/2
  [VVMC_EstSlope_Deg] -> MTQD_RL1TqMapDComp_Z_Nm/1
  [VVMC_EstSlope_Deg] -> MTQD_RL2TqMapDComp_Z_Nm/1
  [VTQD_TqTargetShaftSpd_rpm] -> MTQD_RL2TqMapDComp_Z_Nm/2
  [VTQD_TqTargetShaftSpd_rpm] -> MTQD_RL3TqMapDComp_Z_Nm/2
  [VVMC_EstSlope_Deg] -> MTQD_RL3TqMapDComp_Z_Nm/1
  [VVMC_EstSlope_Deg] -> MTQD_RL4TqMapDComp_Z_Nm/1
  [VTQD_TqTargetShaftSpd_rpm] -> MTQD_RL4TqMapDComp_Z_Nm/2
  [VTQD_TqTargetShaftSpd_rpm] -> MTQD_RL5TqMapDComp_Z_Nm/2
  [VVMC_EstSlope_Deg] -> MTQD_RL5TqMapDComp_Z_Nm/1
  [VTQD_RL1TqMapDComp_Nm] -> Bus Creator/1
  [VTQD_RL2TqMapDComp_Nm] -> Bus Creator/2
  [VTQD_RL3TqMapDComp_Nm] -> Bus Creator/3
  [VTQD_RL4TqMapDComp_Nm] -> Bus Creator/4
  [VTQD_RL5TqMapDComp_Nm] -> Bus Creator/5
  Bus Creator/1 -> [RegenTqMapDComp_bus]  "RegenTqMapDComp_bus"
  [RegenTqMapDComp_bus] -> LUT_D_Normal/11(RegenTqMapDComp_bus)
  [RegenTqMapDComp_bus] -> LUT_D_ECO/13(RegenTqMapDComp_bus)
  [RegenTqMapDComp_bus] -> LUT_D_Sport/11(RegenTqMapDComp_bus)
  VTQD_CreepEnable_flg/1 -> [VTQD_CreepEnable_flg]
  VTQD_BrkSwSta_flg/1 -> [VTQD_BrkSwSta_flg]
  MTQD_RL5TqMapDComp_Z_Nm/1 -> Switch/3
  Switch/1 -> [VTQD_RL5TqMapDComp_Nm]  "VTQD_RL5TqMapDComp_Nm"
  AND/1 -> Switch/2
  [VTQD_BrkSwSta_flg] -> AND/1
  NOT/1 -> AND/2
  Constant/1 -> Switch/1
  Constant1/1 -> Switch1/1
  NOT1/1 -> AND1/2
  AND1/1 -> Switch1/2
  [VTQD_BrkSwSta_flg] -> AND1/1
  MTQD_RL4TqMapDComp_Z_Nm/1 -> Switch1/3
  Switch1/1 -> [VTQD_RL4TqMapDComp_Nm]  "VTQD_RL4TqMapDComp_Nm"
  AND2/1 -> Switch2/2
  NOT2/1 -> AND2/2
  [VTQD_CreepEnable_flg] -> Delay2/1
  Constant2/1 -> Switch2/1
  [VTQD_BrkSwSta_flg] -> AND2/1
  MTQD_RL3TqMapDComp_Z_Nm/1 -> Switch2/3
  Switch2/1 -> [VTQD_RL3TqMapDComp_Nm]  "VTQD_RL3TqMapDComp_Nm"
  AND3/1 -> Switch3/2
  NOT3/1 -> AND3/2
  Constant3/1 -> Switch3/1
  [VTQD_BrkSwSta_flg] -> AND3/1
  MTQD_RL2TqMapDComp_Z_Nm/1 -> Switch3/3
  Switch3/1 -> [VTQD_RL2TqMapDComp_Nm]  "VTQD_RL2TqMapDComp_Nm"
  AND4/1 -> Switch4/2
  NOT4/1 -> AND4/2
  Constant4/1 -> Switch4/1
  [VTQD_BrkSwSta_flg] -> AND4/1
  MTQD_RL1TqMapDComp_Z_Nm/1 -> Switch4/3
  Switch4/1 -> [VTQD_RL1TqMapDComp_Nm]  "VTQD_RL1TqMapDComp_Nm"
  [VTQD_CreepEnable_flg] -> Delay/1
  Delay/1 -> NOT4/1
  [VTQD_CreepEnable_flg] -> Delay1/1
  Delay1/1 -> NOT3/1
  Delay2/1 -> NOT2/1
  [VTQD_CreepEnable_flg] -> Delay3/1
  Delay3/1 -> NOT1/1
  Delay4/1 -> NOT/1
  [VTQD_CreepEnable_flg] -> Delay4/1

== system tqd/TQD/TorqueDemand/TorqueModule/DriverWhlTqDem/PedalMapWhlTq/NoLHM/ShiftPorN ==
  Action Port : ActionPort
  Constant : Constant  Value=ZERO_FLOAT
  VTQD_PedalMapWhlTqPorN_Nm : Outport
  wires:
  Constant/1 -> VTQD_PedalMapWhlTqPorN_Nm/1

== system tqd/TQD/TorqueDemand/TorqueModule/DriverWhlTqDem/PedalMapWhlTq/NoLHM/ShiftR ==
  VTQD_ActAPSPosn_pct : Inport
  VTQD_TqTargetShaftSpd_rpm : Inport  Port=2
  Action Port : ActionPort
  MTQD_NRMTqMapR_Z_Nm : Lookup_n-D  BreakpointsForDimension1=ATQD_NL1TqMapD_Y_pct  BreakpointsForDimension2=ATQD_NL1TqMapD_X_rpm  Table=MTQD_NRMTqMapR_Z_Nm  ExtrapMethod=Clip  InternalRulePriority=Speed  RndMeth=Simplest  InputSameDT=on
      settings: InputPortMap=u0,u1
  VTQD_PedalMapWhlTqR_Nm : Outport
  wires:
  [VTQD_NRMTqMapR_Nm] -> VTQD_PedalMapWhlTqR_Nm/1
  MTQD_NRMTqMapR_Z_Nm/1 -> [VTQD_NRMTqMapR_Nm]
  [VTQD_ActAPSPosn_pct] -> MTQD_NRMTqMapR_Z_Nm/1
  [VTQD_TqTargetShaftSpd_rpm] -> MTQD_NRMTqMapR_Z_Nm/2
  VTQD_ActAPSPosn_pct/1 -> [VTQD_ActAPSPosn_pct]
  VTQD_TqTargetShaftSpd_rpm/1 -> [VTQD_TqTargetShaftSpd_rpm]

== system tqd/TQD/TorqueDemand/TorqueModule/DriverWhlTqDem/PedalMapWhlTq/Pedal G-Control Mode/Active Determination ==
  VINP_SCPSystemMode_enum : Inport
  VPMM_PwrSta_enum : Inport  Port=2
  VTQD_GearActualPosn_enum : Inport  Port=3
  VTQD_RegenMode_enum : Inport  Port=4
  VINP_SWC2RCustomizeSta_flg : Inport  Port=5
  task_time_s : Inport  Port=6
  VINP_SWCResUpSta_flg : Inport  Port=7
  AND : Logic  Inputs=4  AllPortsSameDT=off  OutDataTypeStr=boolean
  AND1 : Logic  AllPortsSameDT=off  OutDataTypeStr=boolean
  AND2 : Logic  AllPortsSameDT=off  OutDataTypeStr=boolean
  AND3 : Logic  AllPortsSameDT=off  OutDataTypeStr=boolean
  AND4 : Logic  Inputs=3  AllPortsSameDT=off  OutDataTypeStr=boolean
  Constant1 : Constant  Value=ENUM_SYSMODE_ENGINEERING
  Constant10 : Constant  Value=ENUM_GEARACTUALPOSN_R
  Constant11 : Constant  Value=KTQD_PedAccTqEn_flg_ovrdflg
  Constant12 : Constant  Value=KTQD_PedGControlModeSW_flg
  Constant13 : Constant  Value=KTQD_PedAccTqEn_flg_ovrdval
  Constant2 : Constant  Value=ENUM_POWERSTA_READY
  Constant21 : Constant  Value=ENUM_SYSMODE_DEVELOPING
  Constant3 : Constant  Value=ENUM_GEARACTUALPOSN_R
  Constant4 : Constant  Value=ENUM_REGENLEVEL_OPD
  Constant5 : Constant  Value=KTQD_PedGControlModeSW_flg
  Constant6 : Constant  Value=KTQD_PedGControlTrigTime_s
  Constant7 : Constant  Value=ENUM_SYSMODE_ENGINEERING
  Constant8 : Constant  Value=ENUM_POWERSTA_READY
  Constant9 : Constant  Value=ENUM_SYSMODE_DEVELOPING
  Delay : Delay  DelayLength=1
  DelayEnable3 : hcu_lib/Basic_Blocks/DelayEnable
  Detect Decrease : simulink/Logic and Bit Operations/Detect Decrease  vinit=0.0  OutDataTypeStr=boolean
  Detect Decrease5 : simulink/Logic and Bit Operations/Detect Decrease  vinit=0.0  OutDataTypeStr=boolean
  Equal{,1..2,4..7} (7 alike) : RelationalOperator  Operator===  OutDataTypeStr=boolean  RndMeth=Simplest
  Equal3 : RelationalOperator  Operator=~=  OutDataTypeStr=boolean  RndMeth=Simplest
  Equal8 : RelationalOperator  Operator=~=  OutDataTypeStr=boolean  RndMeth=Simplest
  OR : Logic  Operator=OR  Inputs=3  AllPortsSameDT=off  OutDataTypeStr=boolean
  OR1 : Logic  Operator=OR  Inputs=3  AllPortsSameDT=off  OutDataTypeStr=boolean
  OR2 : Logic  Operator=OR  AllPortsSameDT=off  OutDataTypeStr=boolean
  OR3 : Logic  Operator=OR  AllPortsSameDT=off  OutDataTypeStr=boolean
  SR_Latch3 : hcu_lib/Basic_Blocks/SR_Latch
  Switch : Switch  Criteria=u2 > Threshold
  VTQD_PedAccTqEn_flg : Outport
  wires:
  Constant2/1 -> Equal2/2
  Constant5/1 -> OR/3
  Constant21/1 -> Equal/2
  Constant1/1 -> Equal1/2
  Equal2/1 -> AND/2
  [VINP_SCPSystemMode_enum] -> Equal1/1
  Equal1/1 -> OR/2
  [VTQD_GearActualPosn_enum] -> Equal3/1
  Equal4/1 -> AND/4
  Constant3/1 -> Equal3/2
  Equal3/1 -> AND/3
  [VPMM_PwrSta_enum] -> Equal2/1
  Equal/1 -> OR/1
  Constant4/1 -> Equal4/2
  OR/1 -> AND/1
  [VTQD_RegenMode_enum] -> Equal4/1
  AND/1 -> [VTQD_PedGControlAllow_flg]  "VTQD_PedGControlAllow_flg"
  [VINP_SCPSystemMode_enum] -> Equal/1
  Detect Decrease5/1 -> AND1/1, SR_Latch3/1
  Delay/1 -> AND1/2
  Constant6/1 -> DelayEnable3/2
  [task_time_s] -> DelayEnable3/3
  DelayEnable3/1 -> Detect Decrease5/1  "VTQD_PedGControlTrig_flg"
  SR_Latch3/1 -> AND2/1
  [VTQD_PedAccTqOperate_flg] -> AND2/2
  [VTQD_PedAccTqEn_flg] -> Delay/1
  VINP_SCPSystemMode_enum/1 -> [VINP_SCPSystemMode_enum]
  VPMM_PwrSta_enum/1 -> [VPMM_PwrSta_enum]
  VTQD_GearActualPosn_enum/1 -> [VTQD_GearActualPosn_enum]
  VTQD_RegenMode_enum/1 -> [VTQD_RegenMode_enum]
  VINP_SWC2RCustomizeSta_flg/1 -> [VINP_SWC2RCustomizeSta_flg]
  task_time_s/1 -> [task_time_s]
  [VTQD_PedAccTqEn_flg] -> VTQD_PedAccTqEn_flg/1
  [VTQD_PedGControlAllow_flg] -> AND3/1
  AND3/1 -> DelayEnable3/1
  [VINP_SCPSystemMode_enum] -> Equal5/1
  OR1/1 -> [VTQD_PedGControlModeSW_flg], AND4/1  "VTQD_PedGControlModeSW_flg"
  Equal5/1 -> OR1/1
  [VPMM_PwrSta_enum] -> Equal7/1
  Equal8/1 -> AND4/3
  Constant10/1 -> Equal8/2
  [VTQD_GearActualPosn_enum] -> Equal8/1
  Equal6/1 -> OR1/2
  [VINP_SCPSystemMode_enum] -> Equal6/1
  Equal7/1 -> AND4/2
  Constant7/1 -> Equal6/2
  Constant9/1 -> Equal5/2
  Constant12/1 -> OR1/3
  Constant8/1 -> Equal7/2
  AND4/1 -> [VTQD_PedAccTqOperate_flg]  "VTQD_PedAccTqOperate_flg"
  AND1/1 -> OR2/1
  OR2/1 -> SR_Latch3/2
  Detect Decrease/1 -> OR2/2
  [VTQD_PedGControlModeSW_flg] -> Detect Decrease/1
  AND2/1 -> Switch/3
  Switch/1 -> [VTQD_PedAccTqEn_flg]  "VTQD_PedAccTqEn_flg"
  Constant11/1 -> Switch/2
  Constant13/1 -> Switch/1
  VINP_SWCResUpSta_flg/1 -> [VINP_SWCResUpSta_flg]
  OR3/1 -> AND3/2
  [VINP_SWC2RCustomizeSta_flg] -> OR3/1
  [VINP_SWCResUpSta_flg] -> OR3/2
